simulink model "MOTOR2015RC_modify2"  (Simulink 10.2)
settings: Solver=VariableStepAuto  StartTime=0.0  StopTime=10  MaxStep=0.000001  RelTol=1e-3  EnableMultiTasking=on
model workspace (MAT data in the model file):
  Ld = 0.0045
  Lq = 0.0085
  Ls = 0.0085
  Rs : num (value not decoded)
undefined symbols (not defined in the file): DiscIntNeverNeededParam
libraries: powerlib x4, pid_lib x4, simulink x1, powerlib_meascontrol x1
settings Model: Creator=Dell  LastModifiedBy=ChenZhi  OrderedModelArguments=off
settings DataIOCC: SaveFormat=Dataset  SignalLoggingSaveFormat=Dataset
settings DebuggingCC: UnderspecifiedInitializationDetection=Simplified  MergeDetectMultiDrivingBlocksExec=error  MaxConsecutiveZCsMsg=none  FcnCallInpInsideContextMsg=error  AllowSymbolicDim=off
settings HardwareCC: ProdBitPerPointer=64  ProdLargestAtomicFloat=Float  ProdIntDivRoundTo=Zero  ProdEndianess=LittleEndian  ProdHWDeviceType=Specified
settings ModelReferenceCC: PropagateSignalLabelsOutOfModel=on
settings GRTTargetCC: CombineOutputUpdateFcns=on  GRTInterface=off
settings SimscapeCC: SimscapeNormalizeSystem=off

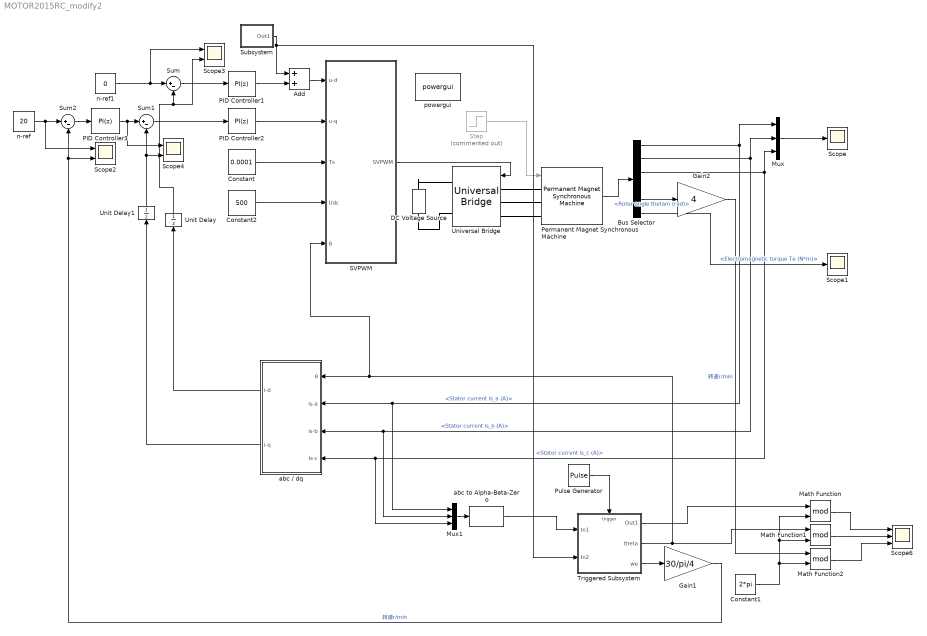
== system MOTOR2015RC_modify2 ==
  Add : Sum
  Bus Selector : BusSelector  OutputSignals=Stator current is_a (A),Stator current is_b (A),Stator current is_c (A),Rotor speed wm (rad/s),Rotor angle thetam (rad),Electromagnetic torque Te (N*m)
  Constant : Constant  Value=0.0001
  Constant1 : Constant  Value=2*pi
  Constant2 : Constant  Value=500
  DC Voltage Source : powerlib/Electrical Sources/DC Voltage Source  Amplitude=500  Measurements=None
  Gain1 : Gain  Gain=30/pi/4
  Gain2 : Gain  Gain=4
  Math Function : Math  Operator=mod  SaturateOnIntegerOverflow=on
  Math Function1 : Math  Operator=mod  SaturateOnIntegerOverflow=on
  Math Function2 : Math  Operator=mod  SaturateOnIntegerOverflow=on
  Mux : Mux  Inputs=3
  Mux1 : Mux  Inputs=3
  PID Controller1 : pid_lib/PID Controller  Controller=PI  Form=Parallel  TimeDomain=Discrete-time  UseExternalTs=off  SampleTime=0.0001  IntegratorMethod=Forward Euler  FilterMethod=Forward Euler  ControllerParametersSource=internal  P=Ls*500*pi  I=Rs*500*pi  D=0  UseFilter=on  N=100  TunerSelectOption=Transfer Function Based (PID Tuner App)  InitialConditionSource=internal  InitialConditionForIntegrator=0  InitialConditionForFilter=0  DifferentiatorICPrevScaledInput=0  ExternalReset=none  TrackingMode=off  Kt=1  LimitOutput=on  SatLimitsSource=internal  UpperSaturationLimit=1000  LowerSaturationLimit=-1000  LinearizeAsGain=on  AntiWindupMode=none  Kb=1  POutMin=[]  POutMax=[]  IOutMin=[]  IOutMax=[]  DOutMin=[]  DOutMax=[]  NOutMin=[]  NOutMax=[]  SumOutMin=[]  SumOutMax=[]  SaturationOutMin=[]  SaturationOutMax=[]  PParamMin=[]  PParamMax=[]  IParamMin=[]  IParamMax=[]  DParamMin=[]  DParamMax=[]  NParamMin=[]  NParamMax=[]  KbParamMin=[]  KbParamMax=[]  KtParamMin=[]  KtParamMax=[]  KbOutMin=[]  KbOutMax=[]  KtOutMin=[]  KtOutMax=[]  IntegratorOutMin=[]  IntegratorOutMax=[]  FilterOutMin=[]  FilterOutMax=[]  SumI1OutMin=[]  SumI1OutMax=[]  SumI2OutMin=[]  SumI2OutMax=[]  SumI3OutMin=[]  SumI3OutMax=[]  SumI4OutMin=[]  SumI4OutMax=[]  SumDOutMin=[]  SumDOutMax=[]  DifferentiatorOutMin=[]  DifferentiatorOutMax=[]  FilterDiffOutCoefMin=[]  FilterDiffOutCoefMax=[]  ReciprocalOutMin=[]  ReciprocalOutMax=[]  SumDenOutMin=[]  SumDenOutMax=[]  SumNumOutMin=[]  SumNumOutMax=[]  DivideOutMin=[]  DivideOutMax=[]  UdiffTsProdOutMin=[]  UdiffTsProdOutMax=[]  NTsProdOutMin=[]  NTsProdOutMax=[]  UintegralTsProdOutMin=[]  UintegralTsProdOutMax=[]  UngainTsProdOutMin=[]  UngainTsProdOutMax=[]  IntegratorContinuousStateAttributes=''  IntegratorStateMustResolveToSignalObject=off  IntegratorRTWStateStorageClass=Auto  FilterContinuousStateAttributes=''  FilterStateMustResolveToSignalObject=off  FilterRTWStateStorageClass=Auto  ParallelPVariant=InternalParameters  IdealPVariant=Disabled  IVariant=InternalParameters  DVariant=Disabled  IntegratorVariant=Discrete  SatVariant=Enabled  AWVariant=Passthrough  PCopyVariant=Disabled  TRVariant=Disabled  FdbkBlocksVariant=Forward  IdealPFdbkVariant=Disabled  SatFdbkVariant=Disabled  DerivativeFilterVariant=Disabled  NVariant=Disabled  NCopyVariant=Disabled_SignalSpec  FilterICVariant=Disabled  IntegratorICVariant=InternalICs  ExternalResetVariant=Disabled  TRSumVariant=Passthrough  SumFdbkVariant=Disabled  SumVariant=Sum_PI  TsampFilterVariant=InternalTs  TsampNgainVariant=Passthrough  TsampIntegralVariant=Passthrough  ExternalSaturationOutDataTypeStr=Inherit: Same as second input
  PID Controller2 : pid_lib/PID Controller  Controller=PI  Form=Parallel  TimeDomain=Discrete-time  UseExternalTs=off  SampleTime=0.0001  IntegratorMethod=Forward Euler  FilterMethod=Forward Euler  ControllerParametersSource=internal  P=Ls*500*pi  I=Rs*500*pi  D=0  UseFilter=on  N=100  TunerSelectOption=Transfer Function Based (PID Tuner App)  InitialConditionSource=internal  InitialConditionForIntegrator=0  InitialConditionForFilter=0  DifferentiatorICPrevScaledInput=0  ExternalReset=none  TrackingMode=off  Kt=1  LimitOutput=on  SatLimitsSource=internal  UpperSaturationLimit=1000  LowerSaturationLimit=-1000  LinearizeAsGain=on  AntiWindupMode=none  Kb=1  POutMin=[]  POutMax=[]  IOutMin=[]  IOutMax=[]  DOutMin=[]  DOutMax=[]  NOutMin=[]  NOutMax=[]  SumOutMin=[]  SumOutMax=[]  SaturationOutMin=[]  SaturationOutMax=[]  PParamMin=[]  PParamMax=[]  IParamMin=[]  IParamMax=[]  DParamMin=[]  DParamMax=[]  NParamMin=[]  NParamMax=[]  KbParamMin=[]  KbParamMax=[]  KtParamMin=[]  KtParamMax=[]  KbOutMin=[]  KbOutMax=[]  KtOutMin=[]  KtOutMax=[]  IntegratorOutMin=[]  IntegratorOutMax=[]  FilterOutMin=[]  FilterOutMax=[]  SumI1OutMin=[]  SumI1OutMax=[]  SumI2OutMin=[]  SumI2OutMax=[]  SumI3OutMin=[]  SumI3OutMax=[]  SumI4OutMin=[]  SumI4OutMax=[]  SumDOutMin=[]  SumDOutMax=[]  DifferentiatorOutMin=[]  DifferentiatorOutMax=[]  FilterDiffOutCoefMin=[]  FilterDiffOutCoefMax=[]  ReciprocalOutMin=[]  ReciprocalOutMax=[]  SumDenOutMin=[]  SumDenOutMax=[]  SumNumOutMin=[]  SumNumOutMax=[]  DivideOutMin=[]  DivideOutMax=[]  UdiffTsProdOutMin=[]  UdiffTsProdOutMax=[]  NTsProdOutMin=[]  NTsProdOutMax=[]  UintegralTsProdOutMin=[]  UintegralTsProdOutMax=[]  UngainTsProdOutMin=[]  UngainTsProdOutMax=[]  IntegratorContinuousStateAttributes=''  IntegratorStateMustResolveToSignalObject=off  IntegratorRTWStateStorageClass=Auto  FilterContinuousStateAttributes=''  FilterStateMustResolveToSignalObject=off  FilterRTWStateStorageClass=Auto  ParallelPVariant=InternalParameters  IdealPVariant=Disabled  IVariant=InternalParameters  DVariant=Disabled  IntegratorVariant=Discrete  SatVariant=Enabled  AWVariant=Passthrough  PCopyVariant=Disabled  TRVariant=Disabled  FdbkBlocksVariant=Forward  IdealPFdbkVariant=Disabled  SatFdbkVariant=Disabled  DerivativeFilterVariant=Disabled  NVariant=Disabled  NCopyVariant=Disabled_SignalSpec  FilterICVariant=Disabled  IntegratorICVariant=InternalICs  ExternalResetVariant=Disabled  TRSumVariant=Passthrough  SumFdbkVariant=Disabled  SumVariant=Sum_PI  TsampFilterVariant=InternalTs  TsampNgainVariant=Passthrough  TsampIntegralVariant=Passthrough  ExternalSaturationOutDataTypeStr=Inherit: Same as second input
  PID Controller3 : pid_lib/PID Controller  Controller=PI  Form=Parallel  TimeDomain=Discrete-time  UseExternalTs=off  SampleTime=0.001  IntegratorMethod=Forward Euler  FilterMethod=Forward Euler  ControllerParametersSource=internal  P=0.1  I=0.01  D=0  UseFilter=on  N=100  TunerSelectOption=Transfer Function Based (PID Tuner App)  InitialConditionSource=internal  InitialConditionForIntegrator=0  InitialConditionForFilter=0  DifferentiatorICPrevScaledInput=0  ExternalReset=none  TrackingMode=off  Kt=1  LimitOutput=on  SatLimitsSource=internal  UpperSaturationLimit=1500  LowerSaturationLimit=-1500  LinearizeAsGain=on  AntiWindupMode=none  Kb=1  POutMin=[]  POutMax=[]  IOutMin=[]  IOutMax=[]  DOutMin=[]  DOutMax=[]  NOutMin=[]  NOutMax=[]  SumOutMin=[]  SumOutMax=[]  SaturationOutMin=[]  SaturationOutMax=[]  PParamMin=[]  PParamMax=[]  IParamMin=[]  IParamMax=[]  DParamMin=[]  DParamMax=[]  NParamMin=[]  NParamMax=[]  KbParamMin=[]  KbParamMax=[]  KtParamMin=[]  KtParamMax=[]  KbOutMin=[]  KbOutMax=[]  KtOutMin=[]  KtOutMax=[]  IntegratorOutMin=[]  IntegratorOutMax=[]  FilterOutMin=[]  FilterOutMax=[]  SumI1OutMin=[]  SumI1OutMax=[]  SumI2OutMin=[]  SumI2OutMax=[]  SumI3OutMin=[]  SumI3OutMax=[]  SumI4OutMin=[]  SumI4OutMax=[]  SumDOutMin=[]  SumDOutMax=[]  DifferentiatorOutMin=[]  DifferentiatorOutMax=[]  FilterDiffOutCoefMin=[]  FilterDiffOutCoefMax=[]  ReciprocalOutMin=[]  ReciprocalOutMax=[]  SumDenOutMin=[]  SumDenOutMax=[]  SumNumOutMin=[]  SumNumOutMax=[]  DivideOutMin=[]  DivideOutMax=[]  UdiffTsProdOutMin=[]  UdiffTsProdOutMax=[]  NTsProdOutMin=[]  NTsProdOutMax=[]  UintegralTsProdOutMin=[]  UintegralTsProdOutMax=[]  UngainTsProdOutMin=[]  UngainTsProdOutMax=[]  IntegratorContinuousStateAttributes=''  IntegratorStateMustResolveToSignalObject=off  IntegratorRTWStateStorageClass=Auto  FilterContinuousStateAttributes=''  FilterStateMustResolveToSignalObject=off  FilterRTWStateStorageClass=Auto  ParallelPVariant=InternalParameters  IdealPVariant=Disabled  IVariant=InternalParameters  DVariant=Disabled  IntegratorVariant=Discrete  SatVariant=Enabled  AWVariant=Passthrough  PCopyVariant=Disabled  TRVariant=Disabled  FdbkBlocksVariant=Forward  IdealPFdbkVariant=Disabled  SatFdbkVariant=Disabled  DerivativeFilterVariant=Disabled  NVariant=Disabled  NCopyVariant=Disabled_SignalSpec  FilterICVariant=Disabled  IntegratorICVariant=InternalICs  ExternalResetVariant=Disabled  TRSumVariant=Passthrough  SumFdbkVariant=Disabled  SumVariant=Sum_PI  TsampFilterVariant=InternalTs  TsampNgainVariant=Passthrough  TsampIntegralVariant=Passthrough  ExternalSaturationOutDataTypeStr=Inherit: Same as second input
  Permanent Magnet Synchronous Machine : powerlib/Machines/Permanent Magnet Synchronous Machine  NbPhases=3  FluxDistribution=Sinusoidal  RotorType=Salient-pole  MechanicalLoad=Torque Tm  PresetModel=No  ShowDetailedParameters=on  MeasurementBus=off  Resistance=Rs  Inductance=8.5e-3  dqInductances=[Ld,Lq]  La=Ls  MachineConstant=Flux linkage established by magnets (V.s)  Flux=0.175  VoltageCst=126.966  TorqueCst=1.05  Flat=120  Mechanical=[0.008 0.0004924 4 0]  PolePairs=4  InitialConditions=[0,0, 0,0]  InitialConditions5ph=[0 0 0 0 0 0]  RefAngle=Aligned with phase A axis (original Park)  IterativeDiscreteModel=Trapezoidal non iterative  TsBlock=-1  TsPowergui=0
  Pulse Generator : DiscretePulseGenerator  PulseType=Time based  Amplitude=20  Period=0.0001  PulseWidth=50  PhaseDelay=-0.0000001
  SVPWM : Subsystem
  Scope : Scope
  Scope1 : Scope
  Scope2 : Scope  NumInputPorts=2
  Scope3 : Scope  NumInputPorts=2
  Scope4 : Scope  NumInputPorts=2
  Scope6 : Scope  NumInputPorts=3
  Step : Step  Commented=on  Time=0.3  Before=4  After=10  SampleTime=0
  Subsystem : Subsystem
  Sum : Sum  Inputs=|+-
  Sum1 : Sum  Inputs=|+-
  Sum2 : Sum  Inputs=|+-
  Triggered Subsystem : Subsystem  TreatAsAtomicUnit=on  mask{rou=50}
  Unit Delay : UnitDelay  SampleTime=-1  HasFrameUpgradeWarning=on
  Unit Delay1 : UnitDelay  SampleTime=-1  HasFrameUpgradeWarning=on
  Universal Bridge : powerlib/Power Electronics/Universal Bridge  Arms=3  SnubberResistance=1e5  SnubberCapacitance=inf  Device=IGBT / Diodes  Ron=1e-3  Lon=0  ForwardVoltages="[  0  0  ]"  ForwardVoltage=0  GTOparameters=[ 10e-6 , 20e-6 ]  IGBTparameters=[ 1e-6 , 2e-6 ]  Measurements=None  Measurements_2=None  converterType=Rectifier
  abc / dq : Subsystem
  abc to Alpha-Beta-Zero : powerlib_meascontrol/Transformations/abc to Alpha-Beta-Zero
  n-ref : Constant  Value=20
  n-ref1 : Constant  Value=0
  powergui : powerlib/powergui  Priority=1  SimulationMode=Continuous  SampleTime=40e-7  frequency=60  Iterations=50  frequencyindice=0  Pbase=100e6  ErrMax=1e-4  UnitsV=kV  UnitsW=MW  buscounter=0  FunctionMessages=off  echomessages=off  EnableUseOfTLC=off  CurrentSourceSwitches=off  DisableSnubberDevices=off  DisableRonSwitches=off  DisableVfSwitches=off  DisplayEquations=off  AutomaticDiscreteSolvers=off  SolverType=Tustin/Backward Euler (TBE)  Interpol=off  ExternalGateDelay=off  methode=off  Ts=10  x0status=blocks  SPID=off  SwTol=0  HookPort=off  NonlinearTolerance=1e-4  nMaxIteration=100  ContinueOnMaxIteration=off  RestoreLinks=warning  ResistiveCurrentMeasurement=off  Frange=[0:2:500]  Ylog=off  Xlog=on  ShowGrid=off  save=off  variable=ZData  structure=0  ZoomFFT=off  StartTime=0.0  cycles=1  DisplayStyle=1  fundamental=60  FreqAxis=off  MaxFrequency=1000  frequencyindicesteady=1  RmsSteady=1  display=off
  wires:
  Permanent Magnet Synchronous Machine/1 -> Bus Selector/1
  SVPWM/1(SVPWM) -> Universal Bridge/1
  PID Controller1/1 -> Add/2
  PID Controller2/1 -> SVPWM/2(u-q)
  Constant/1 -> SVPWM/3(Ts)
  Constant2/1 -> SVPWM/4(Udc)
  Step/1 -> Permanent Magnet Synchronous Machine/1
  Sum/1 -> PID Controller1/1
  Sum1/1 -> PID Controller2/1
  abc / dq/1(i-d) -> Unit Delay/1
  abc / dq/2(i-q) -> Unit Delay1/1
  PID Controller3/1 -> Scope4/1, Sum1/1
  n-ref1/1 -> Scope3/1, Sum/1
  Bus Selector/1 -> Mux/1, Mux1/1, abc / dq/2(is-a)  "<Stator current is_a (A)>"
  Bus Selector/2 -> Mux/2, Mux1/2, abc / dq/3(is-b)  "<Stator current is_b (A)>"
  Bus Selector/3 -> Mux/3, Mux1/3, abc / dq/4(is-c)  "<Stator current is_c (A)>"
  Gain1/1 -> Scope2/2, Sum2/2  "转速r/min"
  n-ref/1 -> Scope2/1, Sum2/1
  Sum2/1 -> PID Controller3/1
  Mux/1 -> Scope/1
  Bus Selector/6 -> Scope1/1  "<Electromagnetic torque Te (N*m)>"
  Unit Delay/1 -> Scope3/2, Sum/2
  Unit Delay1/1 -> Scope4/2, Sum1/2
  Add/1 -> SVPWM/1(u-d)
  Subsystem/1(Out1) -> Add/1, Triggered Subsystem/2(In2)
  Mux1/1 -> abc to Alpha-Beta-Zero/1
  abc to Alpha-Beta-Zero/1 -> Triggered Subsystem/1(In1)
  Pulse Generator/1 -> Triggered Subsystem/Trigger
  Triggered Subsystem/1(Out1) -> Math Function/1
  Triggered Subsystem/2(theta) -> SVPWM/5(θ), abc / dq/1(θ), Math Function1/1
  Constant1/1 -> Math Function2/2, Math Function1/2, Math Function/2
  Math Function/1 -> Scope6/1
  Math Function1/1 -> Scope6/2
  Math Function2/1 -> Scope6/3
  Triggered Subsystem/3(we) -> Gain1/1
  Bus Selector/5 -> Gain2/1  "<Rotor angle thetam (rad)>"
  Gain2/1 -> Math Function2/1  "转速r/min"
  connections:
  Universal Bridge/LConn1 -- Permanent Magnet Synchronous Machine/LConn1
  Universal Bridge/LConn2 -- Permanent Magnet Synchronous Machine/LConn2
  Universal Bridge/LConn3 -- Permanent Magnet Synchronous Machine/LConn3
  DC Voltage Source/RConn1 -- Universal Bridge/RConn1
  Universal Bridge/RConn2 -- DC Voltage Source/LConn1

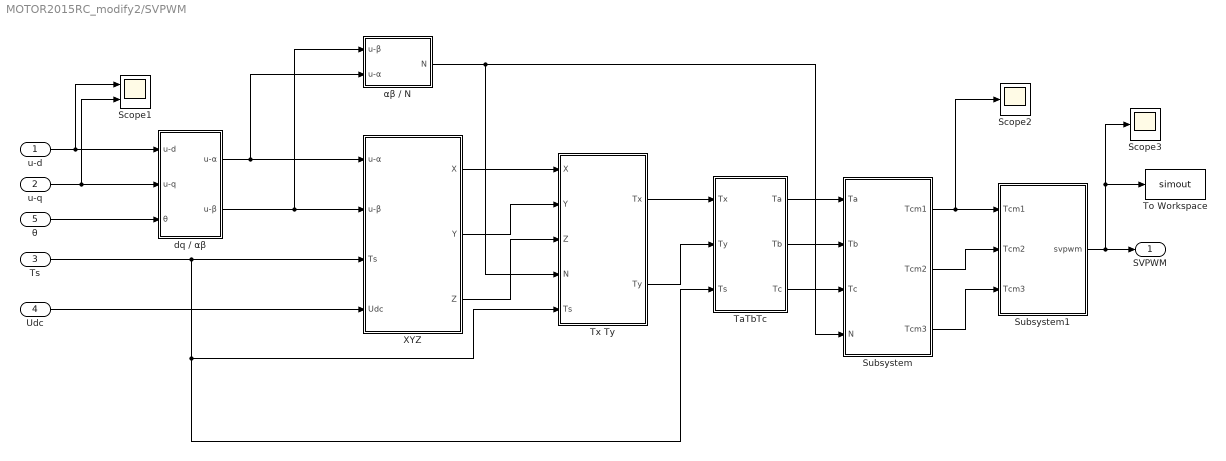
== system MOTOR2015RC_modify2/SVPWM ==
  u-d : Inport
  u-q : Inport  Port=2
  Ts : Inport  Port=3
  Udc : Inport  Port=4
  θ : Inport  Port=5
  Scope1 : Scope  NumInputPorts=2
  Scope2 : Scope
  Scope3 : Scope
  Subsystem : Subsystem
  Subsystem1 : Subsystem
  TaTbTc : Subsystem
  To Workspace : ToWorkspace  VariableName=simout  SaveFormat=Timeseries  SampleTime=-1
  Tx Ty : Subsystem
  XYZ : Subsystem
  dq / αβ : Subsystem
  αβ / N : Subsystem
  SVPWM : Outport  VectorParamsAs1DForOutWhenUnconnected=off
  wires:
  u-d/1 -> Scope1/1, dq / αβ/1(u-d)
  u-q/1 -> Scope1/2, dq / αβ/2(u-q)
  θ/1 -> dq / αβ/3(θ)
  dq / αβ/2(u-β) -> αβ / N/1(u-β), XYZ/2(u-β)
  dq / αβ/1(u-α) -> αβ / N/2(u-α), XYZ/1(u-α)
  Ts/1 -> Tx Ty/5(Ts), TaTbTc/3(Ts), XYZ/3(Ts)
  Udc/1 -> XYZ/4(Udc)
  XYZ/1(X) -> Tx Ty/1(X)
  XYZ/2(Y) -> Tx Ty/2(Y)
  XYZ/3(Z) -> Tx Ty/3(Z)
  αβ / N/1(N) -> Tx Ty/4(N), Subsystem/4(N)
  Tx Ty/1(Tx) -> TaTbTc/1(Tx)
  Tx Ty/2(Ty) -> TaTbTc/2(Ty)
  TaTbTc/1(Ta) -> Subsystem/1(Ta)
  TaTbTc/2(Tb) -> Subsystem/2(Tb)
  TaTbTc/3(Tc) -> Subsystem/3(Tc)
  Subsystem/1(Tcm1) -> Scope2/1, Subsystem1/1(Tcm1)
  Subsystem/2(Tcm2) -> Subsystem1/2(Tcm2)
  Subsystem/3(Tcm3) -> Subsystem1/3(Tcm3)
  Subsystem1/1(svpwm) -> Scope3/1, To Workspace/1, SVPWM/1

== system MOTOR2015RC_modify2/Subsystem ==
  Add : Sum  Inputs=+-
  Constant1 : Constant  Value=10
  Pulse Generator : DiscretePulseGenerator  PulseType=Time based  Amplitude=20  Period=0.0002  PulseWidth=50
  Out1 : Outport
  wires:
  Constant1/1 -> Add/2
  Pulse Generator/1 -> Add/1
  Add/1 -> Out1/1

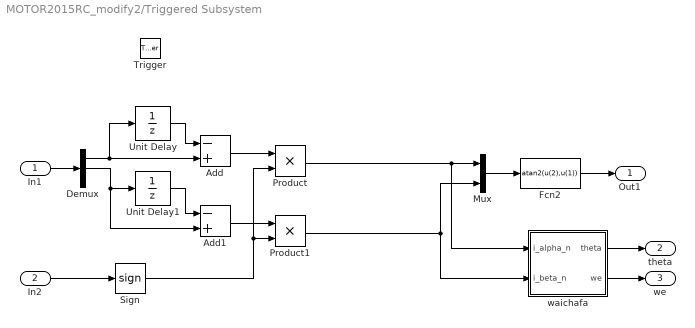
== system MOTOR2015RC_modify2/Triggered Subsystem ==
  In1 : Inport
  In2 : Inport  Port=2
  Trigger : TriggerPort  VariantControl=Variant
  Add : Sum  Inputs=-+
  Add1 : Sum  Inputs=-+
  Demux : Demux  Outputs=3
  Fcn2 : Fcn  Expr=atan2(u(2),u(1))
  Mux : Mux  Inputs=2
  Product : Product
  Product1 : Product
  Sign : Signum
  Unit Delay : UnitDelay  SampleTime=-1  HasFrameUpgradeWarning=on
  Unit Delay1 : UnitDelay  SampleTime=-1  HasFrameUpgradeWarning=on
  waichafa : Subsystem
  Out1 : Outport
  theta : Outport  Port=2
  we : Outport  Port=3
  wires:
  In1/1 -> Demux/1
  Demux/1 -> Add/2, Unit Delay/1
  Unit Delay/1 -> Add/1
  Demux/2 -> Add1/2, Unit Delay1/1
  Unit Delay1/1 -> Add1/1
  Product/1 -> Mux/1, waichafa/1(i_alpha_n)
  Product1/1 -> Mux/2, waichafa/2(i_beta_n)
  Fcn2/1 -> Out1/1
  waichafa/1(theta) -> theta/1
  In2/1 -> Sign/1
  Add/1 -> Product/1
  Sign/1 -> Product1/2, Product/2
  Add1/1 -> Product1/1
  Mux/1 -> Fcn2/1
  waichafa/2(we) -> we/1

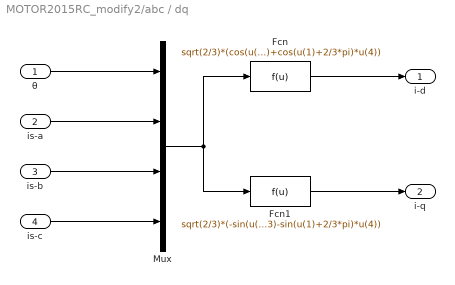
== system MOTOR2015RC_modify2/abc / dq ==
  θ : Inport
  is-a : Inport  Port=2
  is-b : Inport  Port=3
  is-c : Inport  Port=4
  Fcn : Fcn  Expr=sqrt(2/3)*(cos(u(1))*u(2)+cos(u(1)-2/3*pi)*u(3)+cos(u(1)+2/3*pi)*u(4))
  Fcn1 : Fcn  Expr=sqrt(2/3)*(-sin(u(1))*u(2)-sin(u(1)-2/3*pi)*u(3)-sin(u(1)+2/3*pi)*u(4))
  Mux : Mux
  i-d : Outport  VectorParamsAs1DForOutWhenUnconnected=off
  i-q : Outport  Port=2  VectorParamsAs1DForOutWhenUnconnected=off
  wires:
  θ/1 -> Mux/1
  is-a/1 -> Mux/2
  is-b/1 -> Mux/3
  is-c/1 -> Mux/4
  Mux/1 -> Fcn1/1, Fcn/1
  Fcn/1 -> i-d/1
  Fcn1/1 -> i-q/1

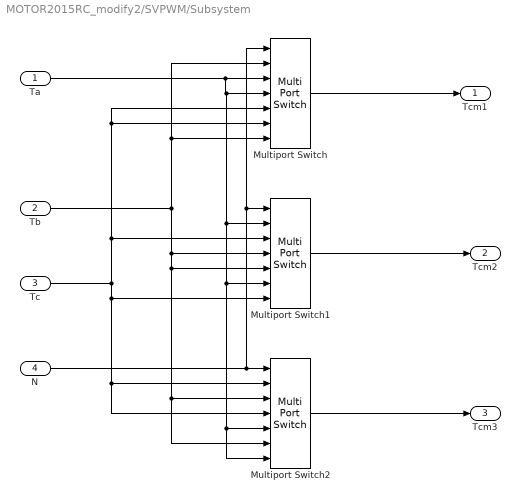
== system MOTOR2015RC_modify2/SVPWM/Subsystem ==
  Ta : Inport
  Tb : Inport  Port=2
  Tc : Inport  Port=3
  N : Inport  Port=4
  Multiport Switch : MultiPortSwitch  Inputs=6
  Multiport Switch1 : MultiPortSwitch  Inputs=6
  Multiport Switch2 : MultiPortSwitch  Inputs=6
  Tcm1 : Outport  VectorParamsAs1DForOutWhenUnconnected=off
  Tcm2 : Outport  Port=2  VectorParamsAs1DForOutWhenUnconnected=off
  Tcm3 : Outport  Port=3  VectorParamsAs1DForOutWhenUnconnected=off
  wires:
  N/1 -> Multiport Switch/1, Multiport Switch1/1, Multiport Switch2/1
  Ta/1 -> Multiport Switch2/7, Multiport Switch2/5, Multiport Switch1/6, Multiport Switch1/2, Multiport Switch/4, Multiport Switch/3
  Tb/1 -> Multiport Switch/7, Multiport Switch/2, Multiport Switch1/5, Multiport Switch2/3, Multiport Switch2/6, Multiport Switch1/4
  Tc/1 -> Multiport Switch1/7, Multiport Switch2/2, Multiport Switch2/4, Multiport Switch1/3, Multiport Switch/5, Multiport Switch/6
  Multiport Switch/1 -> Tcm1/1
  Multiport Switch1/1 -> Tcm2/1
  Multiport Switch2/1 -> Tcm3/1

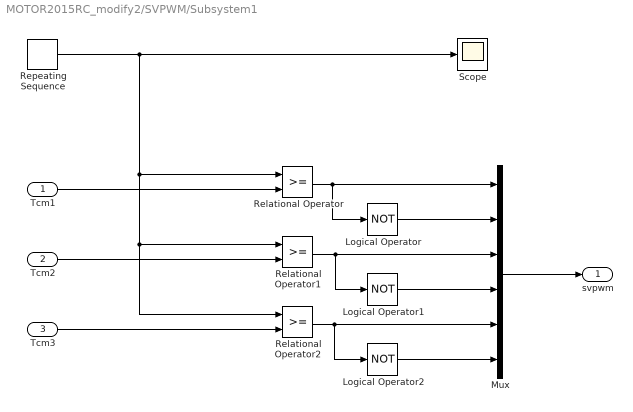
== system MOTOR2015RC_modify2/SVPWM/Subsystem1 ==
  Tcm1 : Inport
  Tcm2 : Inport  Port=2
  Tcm3 : Inport  Port=3
  Logical Operator : Logic  Operator=NOT  AllPortsSameDT=off  OutDataTypeStr=boolean
  Logical Operator1 : Logic  Operator=NOT  AllPortsSameDT=off  OutDataTypeStr=boolean
  Logical Operator2 : Logic  Operator=NOT  AllPortsSameDT=off  OutDataTypeStr=boolean
  Mux : Mux  Inputs=6
  Relational Operator : RelationalOperator  OutDataTypeStr=boolean  ZeroCross=off  RndMeth=Nearest
  Relational Operator1 : RelationalOperator  OutDataTypeStr=boolean  ZeroCross=off  RndMeth=Nearest
  Relational Operator2 : RelationalOperator  OutDataTypeStr=boolean  ZeroCross=off  RndMeth=Nearest
  Repeating Sequence : simulink/Sources/Repeating Sequence  rep_seq_t=[0 0.00005 0.0001]  rep_seq_y=[0 0.00005 0]
  Scope : Scope
  svpwm : Outport  VectorParamsAs1DForOutWhenUnconnected=off
  wires:
  Repeating Sequence/1 -> Relational Operator1/1, Relational Operator2/1, Relational Operator/1, Scope/1
  Tcm1/1 -> Relational Operator/2
  Tcm2/1 -> Relational Operator1/2
  Tcm3/1 -> Relational Operator2/2
  Relational Operator/1 -> Logical Operator/1, Mux/1
  Logical Operator/1 -> Mux/2
  Relational Operator1/1 -> Logical Operator1/1, Mux/3
  Logical Operator1/1 -> Mux/4
  Relational Operator2/1 -> Logical Operator2/1, Mux/5
  Logical Operator2/1 -> Mux/6
  Mux/1 -> svpwm/1

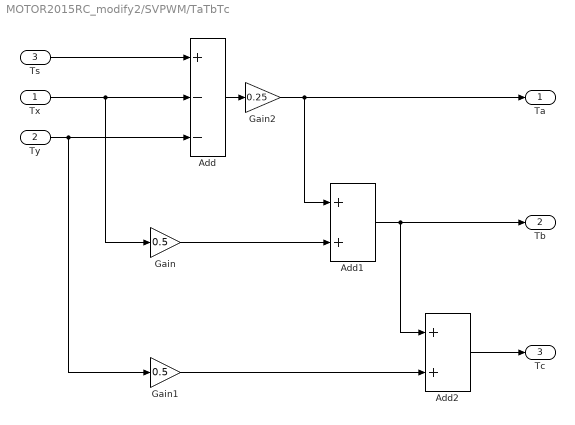
== system MOTOR2015RC_modify2/SVPWM/TaTbTc ==
  Tx : Inport
  Ty : Inport  Port=2
  Ts : Inport  Port=3
  Add : Sum  Inputs=+--
  Add1 : Sum
  Add2 : Sum
  Gain : Gain  Gain=0.5
  Gain1 : Gain  Gain=0.5
  Gain2 : Gain  Gain=0.25
  Ta : Outport  VectorParamsAs1DForOutWhenUnconnected=off
  Tb : Outport  Port=2  VectorParamsAs1DForOutWhenUnconnected=off
  Tc : Outport  Port=3  VectorParamsAs1DForOutWhenUnconnected=off
  wires:
  Ts/1 -> Add/1
  Tx/1 -> Gain/1, Add/2
  Ty/1 -> Gain1/1, Add/3
  Gain/1 -> Add1/2
  Add1/1 -> Add2/1, Tb/1
  Gain1/1 -> Add2/2
  Add2/1 -> Tc/1
  Add/1 -> Gain2/1
  Gain2/1 -> Add1/1, Ta/1

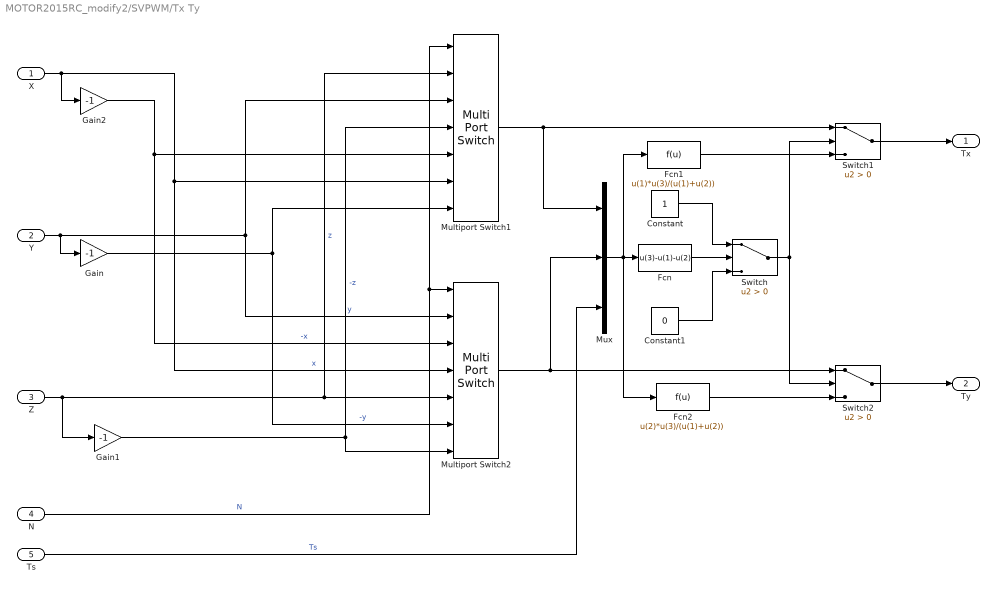
== system MOTOR2015RC_modify2/SVPWM/Tx Ty ==
  X : Inport
  Y : Inport  Port=2
  Z : Inport  Port=3
  N : Inport  Port=4
  Ts : Inport  Port=5
  Constant : Constant
  Constant1 : Constant  Value=0
  Fcn : Fcn  Expr=u(3)-u(1)-u(2)
  Fcn1 : Fcn  Expr=u(1)*u(3)/(u(1)+u(2))
  Fcn2 : Fcn  Expr=u(2)*u(3)/(u(1)+u(2))
  Gain : Gain  Gain=-1
  Gain1 : Gain  Gain=-1
  Gain2 : Gain  Gain=-1
  Multiport Switch1 : MultiPortSwitch  Inputs=6
  Multiport Switch2 : MultiPortSwitch  Inputs=6
  Mux : Mux  Inputs=3
  Switch : Switch  Criteria=u2 > Threshold
  Switch1 : Switch  Criteria=u2 > Threshold
  Switch2 : Switch  Criteria=u2 > Threshold
  Tx : Outport  VectorParamsAs1DForOutWhenUnconnected=off
  Ty : Outport  Port=2  VectorParamsAs1DForOutWhenUnconnected=off
  wires:
  N/1 -> Multiport Switch1/1, Multiport Switch2/1  "N"
  Z/1 -> Multiport Switch1/2, Multiport Switch2/5, Gain1/1  "z"
  Y/1 -> Multiport Switch1/3, Multiport Switch2/2, Gain/1  "y"
  Gain/1 -> Multiport Switch1/7, Multiport Switch2/6  "-y"
  Gain1/1 -> Multiport Switch1/4, Multiport Switch2/7  "-z"
  X/1 -> Gain2/1, Multiport Switch1/6, Multiport Switch2/4  "x"
  Gain2/1 -> Multiport Switch1/5, Multiport Switch2/3  "-x"
  Multiport Switch1/1 -> Switch1/1, Mux/1
  Ts/1 -> Mux/3  "Ts"
  Multiport Switch2/1 -> Mux/2, Switch2/1
  Mux/1 -> Fcn2/1, Fcn1/1, Fcn/1
  Fcn/1 -> Switch/2
  Switch/1 -> Switch1/2, Switch2/2
  Switch1/1 -> Tx/1
  Switch2/1 -> Ty/1
  Fcn1/1 -> Switch1/3
  Fcn2/1 -> Switch2/3
  Constant/1 -> Switch/1
  Constant1/1 -> Switch/3

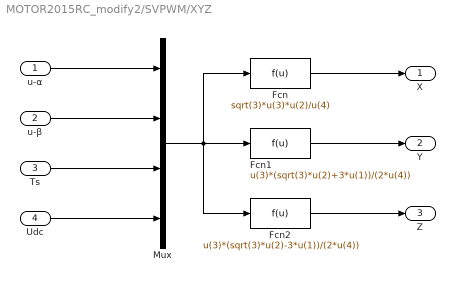
== system MOTOR2015RC_modify2/SVPWM/XYZ ==
  u-α : Inport
  u-β : Inport  Port=2
  Ts : Inport  Port=3
  Udc : Inport  Port=4
  Fcn : Fcn  Expr=sqrt(3)*u(3)*u(2)/u(4)
  Fcn1 : Fcn  Expr=u(3)*(sqrt(3)*u(2)+3*u(1))/(2*u(4))
  Fcn2 : Fcn  Expr=u(3)*(sqrt(3)*u(2)-3*u(1))/(2*u(4))
  Mux : Mux
  X : Outport  VectorParamsAs1DForOutWhenUnconnected=off
  Y : Outport  Port=2  VectorParamsAs1DForOutWhenUnconnected=off
  Z : Outport  Port=3  VectorParamsAs1DForOutWhenUnconnected=off
  wires:
  u-α/1 -> Mux/1
  u-β/1 -> Mux/2
  Ts/1 -> Mux/3
  Udc/1 -> Mux/4
  Mux/1 -> Fcn2/1, Fcn1/1, Fcn/1
  Fcn/1 -> X/1
  Fcn1/1 -> Y/1
  Fcn2/1 -> Z/1

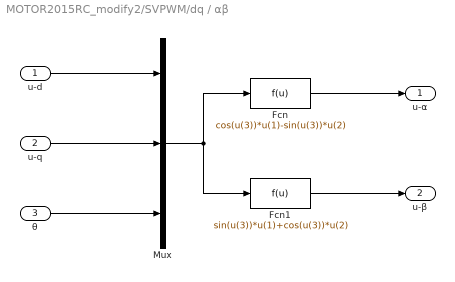
== system MOTOR2015RC_modify2/SVPWM/dq / αβ ==
  u-d : Inport
  u-q : Inport  Port=2
  θ : Inport  Port=3
  Fcn : Fcn  Expr=cos(u(3))*u(1)-sin(u(3))*u(2)
  Fcn1 : Fcn  Expr=sin(u(3))*u(1)+cos(u(3))*u(2)
  Mux : Mux  Inputs=3
  u-α : Outport  VectorParamsAs1DForOutWhenUnconnected=off
  u-β : Outport  Port=2  VectorParamsAs1DForOutWhenUnconnected=off
  wires:
  u-d/1 -> Mux/1
  u-q/1 -> Mux/2
  θ/1 -> Mux/3
  Mux/1 -> Fcn1/1, Fcn/1
  Fcn/1 -> u-α/1
  Fcn1/1 -> u-β/1

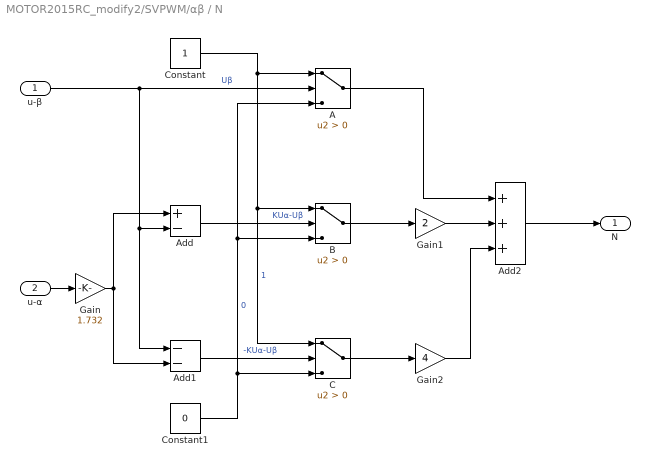
== system MOTOR2015RC_modify2/SVPWM/αβ / N ==
  u-β : Inport
  u-α : Inport  Port=2
  A : Switch  Criteria=u2 > Threshold
  Add : Sum  Inputs=+-
  Add1 : Sum  Inputs=--
  Add2 : Sum  Inputs=+++
  B : Switch  Criteria=u2 > Threshold
  C : Switch  Criteria=u2 > Threshold
  Constant : Constant
  Constant1 : Constant  Value=0
  Gain : Gain  Gain=1.732
  Gain1 : Gain  Gain=2
  Gain2 : Gain  Gain=4
  N : Outport  VectorParamsAs1DForOutWhenUnconnected=off
  wires:
  u-β/1 -> Add1/1, Add/2, A/2  "Uβ"
  Constant/1 -> C/1, B/1, A/1  "1"
  u-α/1 -> Gain/1
  Gain/1 -> Add/1, Add1/2
  Add/1 -> B/2  "KUα-Uβ"
  Constant1/1 -> B/3, A/3, C/3  "0"
  Add1/1 -> C/2  "-KUα-Uβ"
  C/1 -> Gain2/1
  B/1 -> Gain1/1
  A/1 -> Add2/1
  Gain1/1 -> Add2/2
  Gain2/1 -> Add2/3
  Add2/1 -> N/1

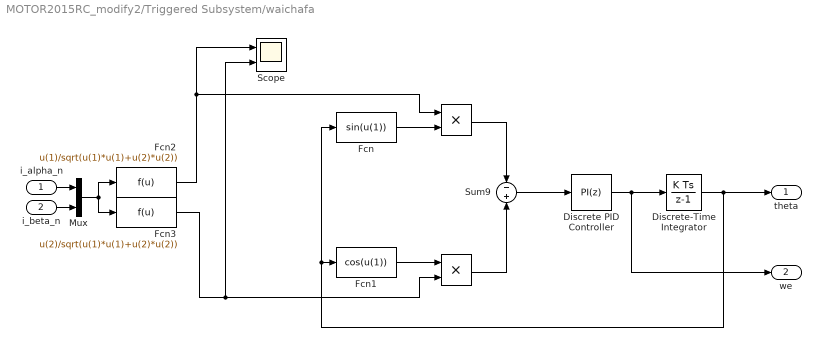
== system MOTOR2015RC_modify2/Triggered Subsystem/waichafa ==
  i_alpha_n : Inport
  i_beta_n : Inport  Port=2
  "   " : Product
  "    " : Product
  Discrete PID Controller : pid_lib/PID Controller  Controller=PI  Form=Parallel  TimeDomain=Discrete-time  UseExternalTs=off  SampleTime=-1  IntegratorMethod=Forward Euler  FilterMethod=Forward Euler  ControllerParametersSource=internal  P=2*rou  I=rou*rou  D=0  UseFilter=on  N=100  TunerSelectOption=Transfer Function Based (PID Tuner App)  InitialConditionSource=internal  InitialConditionForIntegrator=0  InitialConditionForFilter=0  DifferentiatorICPrevScaledInput=0  ExternalReset=none  TrackingMode=off  Kt=1  LimitOutput=off  SatLimitsSource=internal  UpperSaturationLimit=inf  LowerSaturationLimit=-inf  LinearizeAsGain=off  AntiWindupMode=none  Kb=1  POutMin=[]  POutMax=[]  IOutMin=[]  IOutMax=[]  DOutMin=[]  DOutMax=[]  NOutMin=[]  NOutMax=[]  SumOutMin=[]  SumOutMax=[]  SaturationOutMin=[]  SaturationOutMax=[]  PParamMin=[]  PParamMax=[]  IParamMin=[]  IParamMax=[]  DParamMin=[]  DParamMax=[]  NParamMin=[]  NParamMax=[]  KbParamMin=[]  KbParamMax=[]  KtParamMin=[]  KtParamMax=[]  KbOutMin=[]  KbOutMax=[]  KtOutMin=[]  KtOutMax=[]  IntegratorOutMin=[]  IntegratorOutMax=[]  FilterOutMin=[]  FilterOutMax=[]  SumI1OutMin=[]  SumI1OutMax=[]  SumI2OutMin=[]  SumI2OutMax=[]  SumI3OutMin=[]  SumI3OutMax=[]  SumI4OutMin=[]  SumI4OutMax=[]  SumDOutMin=[]  SumDOutMax=[]  DifferentiatorOutMin=[]  DifferentiatorOutMax=[]  FilterDiffOutCoefMin=[]  FilterDiffOutCoefMax=[]  ReciprocalOutMin=[]  ReciprocalOutMax=[]  SumDenOutMin=[]  SumDenOutMax=[]  SumNumOutMin=[]  SumNumOutMax=[]  DivideOutMin=[]  DivideOutMax=[]  UdiffTsProdOutMin=[]  UdiffTsProdOutMax=[]  NTsProdOutMin=[]  NTsProdOutMax=[]  UintegralTsProdOutMin=[]  UintegralTsProdOutMax=[]  UngainTsProdOutMin=[]  UngainTsProdOutMax=[]  IntegratorContinuousStateAttributes=''  IntegratorStateMustResolveToSignalObject=off  IntegratorRTWStateStorageClass=Auto  FilterContinuousStateAttributes=''  FilterStateMustResolveToSignalObject=off  FilterRTWStateStorageClass=Auto  ParallelPVariant=InternalParameters  IdealPVariant=Disabled  IVariant=InternalParameters  DVariant=Disabled  IntegratorVariant=Discrete  SatVariant=Disabled  AWVariant=Passthrough  PCopyVariant=Disabled  TRVariant=Disabled  FdbkBlocksVariant=Forward  IdealPFdbkVariant=Disabled  SatFdbkVariant=Disabled  DerivativeFilterVariant=Disabled  NVariant=Disabled  NCopyVariant=Disabled_SignalSpec  FilterICVariant=Disabled  IntegratorICVariant=InternalICs  ExternalResetVariant=Disabled  TRSumVariant=Passthrough  SumFdbkVariant=Disabled  SumVariant=Sum_PI  TsampFilterVariant=InternalTs  TsampNgainVariant=Passthrough  TsampIntegralVariant=Passthrough  ExternalSaturationOutDataTypeStr=Inherit: Same as second input
  Discrete-Time Integrator : DiscreteIntegrator  SampleTime=-1  ICPrevOutput=DiscIntNeverNeededParam  ICPrevScaledInput=DiscIntNeverNeededParam
  Fcn : Fcn  Expr=sin(u(1))
  Fcn1 : Fcn  Expr=cos(u(1))
  Fcn2 : Fcn  Expr=u(1)/sqrt(u(1)*u(1)+u(2)*u(2))
  Fcn3 : Fcn  Expr=u(2)/sqrt(u(1)*u(1)+u(2)*u(2))
  Mux : Mux  Inputs=2
  Scope : Scope  NumInputPorts=2
  Sum9 : Sum  Inputs=-+
  theta : Outport  VectorParamsAs1DForOutWhenUnconnected=off
  we : Outport  Port=2  VectorParamsAs1DForOutWhenUnconnected=off
  wires:
  "   "/1 -> Sum9/2
  Fcn1/1 -> "   "/1
  "    "/1 -> Sum9/1
  Fcn/1 -> "    "/2
  i_alpha_n/1 -> Mux/1
  Mux/1 -> Fcn3/1, Fcn2/1
  Fcn2/1 -> Scope/1, "    "/1
  Discrete-Time Integrator/1 -> theta/1, Fcn/1, Fcn1/1
  Fcn3/1 -> Scope/2, "   "/2
  Sum9/1 -> Discrete PID Controller/1
  Discrete PID Controller/1 -> we/1, Discrete-Time Integrator/1
  i_beta_n/1 -> Mux/2
